simulink model "single_dmp_test"  (R2020b)
settings: Solver=ode8  StartTime=0.0  StopTime=10.0  FixedStep=0.005  RelTol=1e-3
values from neighbouring files (symbols this model uses):
  cc_new = [1 0.92774349 0.86070798 0.79851622 0.74081822 0.68728928 0.63762815 0.59155536 0.54881164 0.50915642 0.47236655 0.43823499 ... (41 elements, 1x41)]    [my_config_1213.mat]    (also in my_config_1219.mat)
  D = [64.807 64.807 64.807]    [my_config_1213.mat]    (also in my_config_1219.mat)
  K = [1050 1050 1050]    [my_config_1213.mat]    (also in my_config_1219.mat; my_config_1224.mat)
  left_0 = [0 0 0]    [my_config_1219.mat]
  tau1 = 3    [my_config_1213.mat]    (also in my_config_1219.mat)
  weight = [0.0266866854 0.00199886353 0 0.185908993 0.0191898792 0 0.285018336 0.0372844837 0 0.420259935 0.0646488362 0 ... (123 elements, 3x41)]    [my_config_1213.mat]    (also in my_config_1219.mat)
  width_new = [191.53405062 222.53081866 258.54392519 300.38518553 348.99779456 405.47758835 471.09774681 547.33749391 635.91544276 738.82833688 858.39606128 997.31393782 ... (41 elements, 1x41)]    [my_config_1213.mat]    (also in my_config_1219.mat)
settings Model: Creator=10788  LastModifiedBy=10788
settings OptimizationCC: DefaultParameterBehavior=Inlined  UseDivisionForNetSlopeComputation=on  GainParamInheritBuiltInType=on  UseFloatMulNetSlope=on  InlineInvariantSignals=on  PassReuseOutputArgsAs=Individual arguments  ZeroExternalMemoryAtStartup=off  ZeroInternalMemoryAtStartup=off  NoFixptDivByZeroProtection=on  EfficientFloat2IntCast=on  LifeSpan=1  OptimizeBlockOrder=speed  DifferentSizesBufferReuse=on  EfficientTunableParamExpr=on
settings DebuggingCC: ParameterTunabilityLossMsg=error
settings HardwareCC: ProdLongLongMode=on
settings SFSimCC: MATLABDynamicMemAlloc=off  SimTargetLang=C++
settings RTWCC: Description=Embedded Coder  SystemTargetFile=ert.tlc  TemplateMakefile=ert_default_tmf  GenerateReport=on  LaunchReport=on  TargetLang=C++
settings CodeAppCC: ForceParamTrailComments=on  IgnoreCustomStorageClasses=off  OperatorAnnotations=on  SimulinkDataObjDesc=on  SFDataObjDesc=on  CustomSymbolStrGlobalVar=rt$N$M  CustomSymbolStrType=$N$M  CustomSymbolStrFcn=$N$M$F  CustomSymbolStrMacro=$N$M  InsertBlockDesc=on
settings ERTTargetCC: TargetLangStandard=C++03 (ISO)  GenerateSampleERTMain=on  IncludeMdlTerminateFcn=off  CombineSignalStateStructs=on  SupportAbsoluteTime=off  CodeInterfacePackaging=C++ class  SupportComplex=off  SupportContinuousTime=on  SupportNonInlinedSFcns=on  InlinedParameterPlacement=NonHierarchical  RootIOFormat=Structure reference  ERTCustomFileTemplate=example_file_process.tlc  ERTFilePackagingFormat=CompactWithDataFile

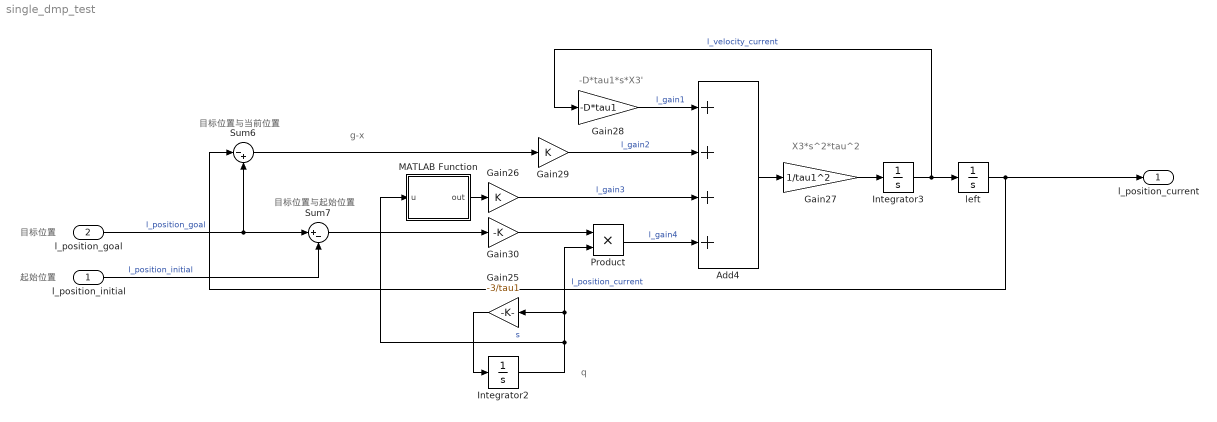
== system single_dmp_test ==
  note: 目标位置与当前位置
  note: 起始位置
  note: X3*s^2*tau^2
  note: 目标位置
  note: 目标位置与起始位置
  note: -D*tau1*s*X3'
  note: g-x
  note: q
  l_position_initial : Inport  OutDataTypeStr=double  PortDimensions=3
  l_position_goal : Inport  Port=2  OutDataTypeStr=double  PortDimensions=3
  Add4 : Sum  Inputs=++++
  Gain25 : Gain  Gain=-3/tau1
  Gain26 : Gain  Gain=K
  Gain27 : Gain  Gain=1/tau1^2
  Gain28 : Gain  Gain=-D*tau1
  Gain29 : Gain  Gain=K
  Gain30 : Gain  Gain=-K
  Integrator2 : Integrator  InitialCondition=1
  Integrator3 : Integrator
  MATLAB Function : MATLAB Function  TreatAsAtomicUnit=on
  Product : Product
  Sum6 : Sum  Inputs=|-+
  Sum7 : Sum  Inputs=|+-
  left : Integrator  InitialCondition=left_0
  l_position_current : Outport
  wires:
  Add4/1 -> Gain27/1
  Product/1 -> Add4/4  "l_gain4"
  Gain25/1 -> Integrator2/1
  Integrator3/1 -> Gain28/1, left/1  "l_velocity_current"
  Gain27/1 -> Integrator3/1
  Sum7/1 -> Gain30/1
  Gain30/1 -> Product/1
  Integrator2/1 -> Product/2, Gain25/1, MATLAB Function/1(u)  "s"
  MATLAB Function/1(out) -> Gain26/1
  Sum6/1 -> Gain29/1
  l_position_goal/1 -> Sum7/1, Sum6/2  "l_position_goal"
  Gain29/1 -> Add4/2  "l_gain2"
  left/1 -> l_position_current/1, Sum6/1  "l_position_current"
  l_position_initial/1 -> Sum7/2  "l_position_initial"
  Gain26/1 -> Add4/3  "l_gain3"
  Gain28/1 -> Add4/1  "l_gain1"

== matlab function single_dmp_test/MATLAB Function ==
  data: u input; out output; width_new parameter; weight parameter; cc_new parameter
function out = fcn(u, width_new, weight, cc_new)


% if(u>2.5)
%     y=1;
% elseif(u>=0&&u<=2.5)
%     y=0;
% else
%         y=-1;
% end


tem=exp(-width_new.*(u-cc_new).^2)';
y=(weight * tem * u) / sum(tem) ;

out = y;
